simulink model "ZweiServer_ZweiWarteschlangen"  (R2017a)
settings: Solver=VariableStepAuto  StartTime=0.0  StopTime=6000  RelTol=1e-3  EnableMultiTasking=on
undefined symbols (not defined in the file): elapsedTime, entity, m, n
settings Model: Creator=gome  LastModifiedBy=Nicolas
settings OptimizationCC: LifeSpan=inf
settings DebuggingCC: SFUnexpectedBacktrackingDiag=warning  SFNoUnconditionalDefaultTransitionDiag=warning  SFExecutionAtInitializationDiag=none
settings GRTTargetCC: TargetLangStandard=C89/C90 (ANSI)  GeneratePreprocessorConditionals=Disable all
settings ConfigComp: CovMetricSettings=dw  CovHtmlReporting=on  CovSaveCumulativeToWorkspaceVar=on  CovSaveSingleToWorkspaceVar=on  CovExternalEMLEnable=off

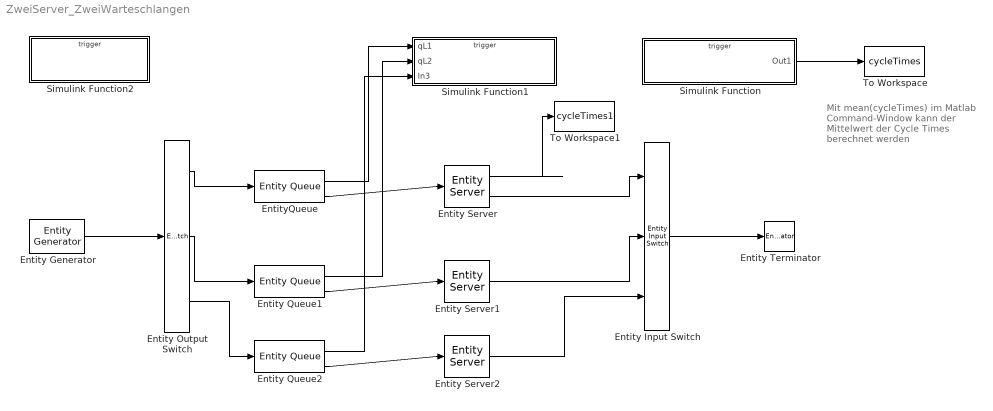
== system ZweiServer_ZweiWarteschlangen ==
  note: Mit mean(cycleTimes) im Matlab Command-Window kann der Mittelwert der Cycle Times berechnet werden
  Entity Input Switch : EntityInputSwitch  InputPortMessageModes=m,m,m  OutputPortMessageModes=m  NumberInputPorts=3
      settings: InputPortMap=u1,u2,u3
  Entity Output Switch : EntityOutputSwitch  InputPortMessageModes=m  OutputPortMessageModes=m,m,m  NumberOutputPorts=3  SwitchingCriterion=From attribute  SwitchAttributeName=portNumber
      settings: OutputPortMap=o0,o1,o2
  Entity Generator : EntityGenerator  OutputPortMessageModes=m  Period=0.5  IntergenerationTimeAction=dt = exprnd(0.5);  GenerateAction=|  AttributeName=portNumber|TimeStamp  AttributeInitialValue=1|1  EntityType=Structured  EntityTypeName=Entity2
      | entity.portNumber = portNumber();
      | entity.TimeStamp = stampEntity();
  Entity Queue1 : EntityQueue  InputPortMessageModes=m  OutputPortMessageModes=n,m  Capacity=inf  NumberEntitiesInBlock=on
      settings: OutputPortMap=o1,o5
  Entity Queue2 : EntityQueue  InputPortMessageModes=m  OutputPortMessageModes=n,m  Capacity=inf  NumberEntitiesInBlock=on
      settings: OutputPortMap=o1,o5
  Entity Server : EntityServer  InputPortMessageModes=m  OutputPortMessageModes=n,m  Capacity=1  ServiceTimeSource=MATLAB action  ServiceTimeAction=dt = exprnd(0.6);  AverageWait=on
      settings: OutputPortMap=o4,o9
  Entity Server1 : EntityServer  InputPortMessageModes=m  OutputPortMessageModes=m  Capacity=1  ServiceTimeSource=MATLAB action  ServiceTimeAction=dt = exprnd(0.6);
  Entity Server2 : EntityServer  InputPortMessageModes=m  OutputPortMessageModes=m  Capacity=1  ServiceTimeSource=MATLAB action  ServiceTimeAction=dt = exprnd(0.6);
  Entity Terminator : EntityTerminator  InputPortMessageModes=m  EntryAction=elapsedTime(entity.TimeStamp);
  EntityQueue : EntityQueue  InputPortMessageModes=m  OutputPortMessageModes=n,m  Capacity=inf  NumberEntitiesInBlock=on
      settings: OutputPortMap=o1,o5
  Simulink Function : Subsystem  TreatAsAtomicUnit=on
  Simulink Function1 : Subsystem  TreatAsAtomicUnit=on
  Simulink Function2 : Subsystem  TreatAsAtomicUnit=on
  To Workspace : ToWorkspace  VariableName=cycleTimes  SampleTime=-1
  To Workspace1 : ToWorkspace  VariableName=cycleTimes1  SampleTime=-1
  wires:
  Entity Generator/1 -> Entity Output Switch/1
  Entity Output Switch/1 -> EntityQueue/1
  Entity Output Switch/2 -> Entity Queue1/1
  EntityQueue/2 -> Entity Server/1
  Entity Queue1/2 -> Entity Server1/1
  Entity Server/2 -> Entity Input Switch/1
  Entity Server1/1 -> Entity Input Switch/2
  Entity Input Switch/1 -> Entity Terminator/1
  EntityQueue/1 -> Simulink Function1/1(qL1)
  Entity Queue1/1 -> Simulink Function1/2(qL2)
  Simulink Function/1(Out1) -> To Workspace/1
  Entity Output Switch/3 -> Entity Queue2/1
  Entity Queue2/1 -> Simulink Function1/3(In3)
  Entity Queue2/2 -> Entity Server2/1
  Entity Server2/1 -> Entity Input Switch/3
  Entity Server/1 -> To Workspace1/1

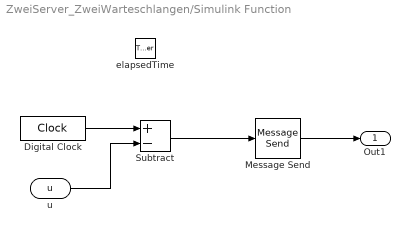
== system ZweiServer_ZweiWarteschlangen/Simulink Function ==
  elapsedTime : TriggerPort  TriggerType=function-call  IsSimulinkFunction=on  FunctionName=elapsedTime  VariantControl=Variant
  Digital Clock : DigitalClock  SampleTime=-1
  Message Send : MessageSend  OutputPortMessageModes=m
      settings: InputPortMap=u1
  Subtract : Sum  Inputs=+-
  u : ArgIn  DisableCoverage=on  ArgumentName=u
  Out1 : Outport
  wires:
  Digital Clock/1 -> Subtract/1
  u/1 -> Subtract/2
  Subtract/1 -> Message Send/1
  Message Send/1 -> Out1/1

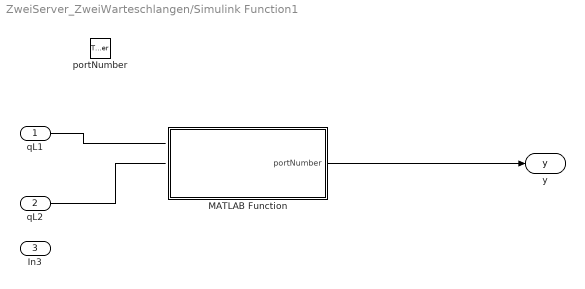
== system ZweiServer_ZweiWarteschlangen/Simulink Function1 ==
  qL1 : Inport
  qL2 : Inport  Port=2
  In3 : Inport  Port=3
  portNumber : TriggerPort  TriggerType=function-call  IsSimulinkFunction=on  FunctionName=portNumber  VariantControl=Variant
  MATLAB Function : MATLAB Function  TreatAsAtomicUnit=on
  y : ArgOut  DisableCoverage=on  ArgumentName=y
  wires:
  qL1/1 -> ?
  qL2/1 -> ?
  MATLAB Function/1(portNumber) -> y/1

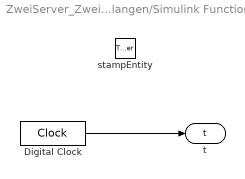
== system ZweiServer_ZweiWarteschlangen/Simulink Function2 ==
  stampEntity : TriggerPort  TriggerType=function-call  IsSimulinkFunction=on  FunctionName=stampEntity  VariantControl=Variant
  Digital Clock : DigitalClock  SampleTime=-1
  t : ArgOut  DisableCoverage=on  ArgumentName=t
  wires:
  Digital Clock/1 -> t/1

== matlab function ZweiServer_ZweiWarteschlangen/Simulink Function1/MATLAB Function ==
  data: portNumber output
function portNumber = fcn()

randN = rand();
if randN < 1/3
    portNumber = 1;
end
if randN > 1/3
    portNumber = 2;
end
if randN < 2/3 && randN > 1/3
    portNumber = 3;
end
